simulink model "assignment3"  (R2020b)
settings: Solver=VariableStepAuto  StartTime=0.0  StopTime=10.0  RelTol=1e-3
undefined symbols (not defined in the file or in its folder): b, Kd, Ki, Kp, m
settings Model: Creator=Sudhanshu  LastModifiedBy=Sudhanshu

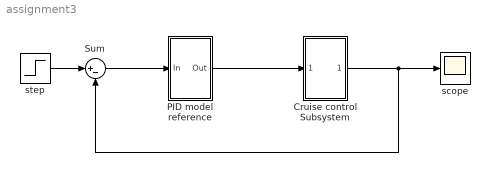
== system assignment3 ==
  Cruise control Subsystem : Subsystem
  PID model reference : Subsystem  TreatAsAtomicUnit=on
  Sum : Sum  Inputs=|+-
  scope : Scope
  step : Step  SampleTime=0
  wires:
  Cruise control Subsystem/1(out) -> scope/1, Sum/2
  step/1 -> Sum/1
  Sum/1 -> PID model reference/1(In)
  PID model reference/1(Out) -> Cruise control Subsystem/1(Inp)

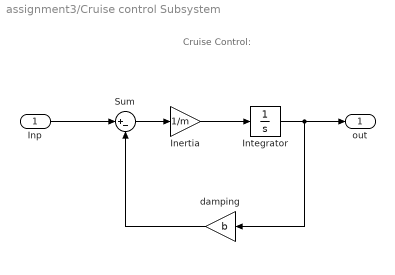
== system assignment3/Cruise control Subsystem ==
  note: Cruise Control:
  Inp : Inport
  Inertia : Gain  Gain=1/m
  Integrator : Integrator
  Sum : Sum  Inputs=|+-
  damping : Gain  Gain=b
  out : Outport
  wires:
  Integrator/1 -> out/1, damping/1
  Inertia/1 -> Integrator/1
  Sum/1 -> Inertia/1
  damping/1 -> Sum/2
  Inp/1 -> Sum/1

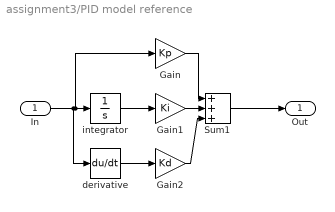
== system assignment3/PID model reference ==
  In : Inport
  Gain : Gain  Gain=Kp
  Gain1 : Gain  Gain=Ki
  Gain2 : Gain  Gain=Kd
  Sum1 : Sum  Inputs=+++
  derivative : Derivative
  integrator : Integrator
  Out : Outport
  wires:
  Gain1/1 -> Sum1/2
  Gain2/1 -> Sum1/3
  Gain/1 -> Sum1/1
  In/1 -> derivative/1, Gain/1, integrator/1
  derivative/1 -> Gain2/1
  integrator/1 -> Gain1/1
  Sum1/1 -> Out/1
